simulink model "RM3_Hydraulic_PTO"  (R2019b)
settings: Solver=ode14x  StartTime=0  StopTime=100  FixedStep=0.0025  MaxStep=0.0025  RelTol=1e-3  EnableMultiTasking=on
undefined symbols (not defined in the file or in its folder): body, DiscIntNeverNeededParam, pto
libraries: fl_lib x208, sh_lib x67, nesl_utility x67, WECSim_Lib x5
(part 2 of 5)

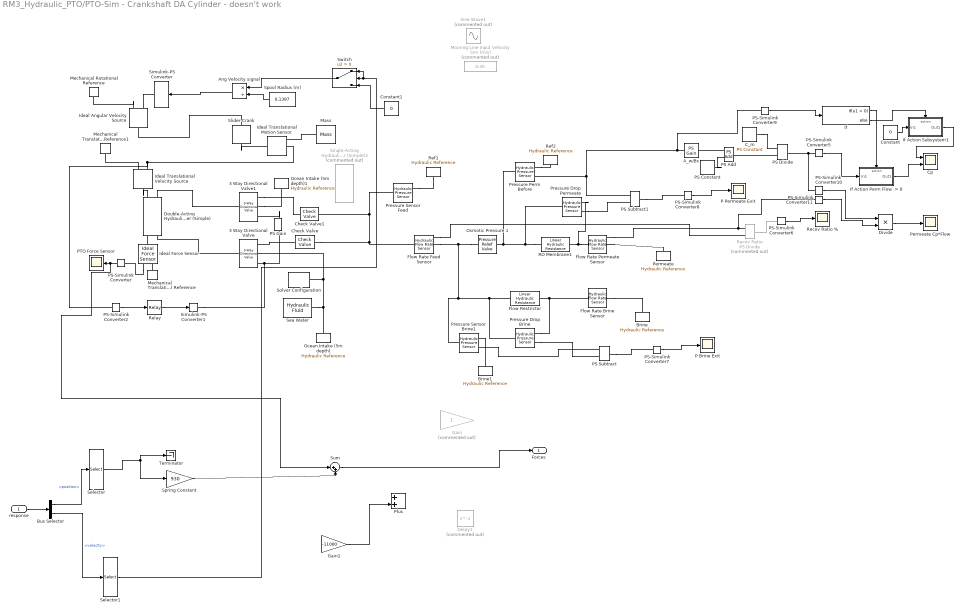
== system RM3_Hydraulic_PTO/PTO-Sim - Crankshaft DA Cylinder - doesn't work ==
  response : Inport
  " Flow Rate Feed Sensor" : fl_lib/Hydraulic/Hydraulic Sensors/Hydraulic Flow Rate Sensor
      settings: SourceProductName=Simscape
  3 Way Directional Valve : sh_lib/Valves/Directional Valves/3-Way Directional Valve  area_spec=sh.valves.directional_valves.enum.area_spec.identical  x_0_P=0 m  x_0_T=0 m  mdl_type_identical=sh.valves.directional_valves.enum.mdl_type.linear  mdl_type_different=sh.valves.directional_valves.enum.mdl_type.linear  opening_max=0.75 in  area_max=pi*(0.75/2)^2 in^2  opening_max_P_A=0.005 m  area_max_P_A=0.5e-4 m^2  opening_max_A_T=0.005 m  area_max_A_T=0.5e-4 m^2  opening_area_tab=[-.002, 0, .002, .005, .015] m  area_tab=[1e-09, 2.0352e-07, 4.0736e-05, .00011438, .00034356] m^2  opening_flow_rate_tab=[-.002, 0, .002, .005, .015] m  pressure_tab=[-10000000, -5000000, -2000000, 2000000, 5000000, 10000000] Pa  flow_rate_tab=[-1e-07, -7.0711e-08, -4.4721e-08, 4.4721e-08, 7.0711e-08, 1e-07; -2.0352e-05, -1.4391e-05, -9.1017e-06, 9.1017e-06, 1.4391e-05, 2.0352e-05; -.0040736, -.0028805, -.0018218, .0018218, .0028805, .0040736; -.011438, -.0080879, -.0051152, .0051152, .0080879, .011438; -.034356, -.024293, -.015364, .015364, .024293, .034356] m^3/s  opening_area_tab_P_A=[-.002, 0, .002, .005, .015] m  area_tab_P_A=[1e-09, 2.0352e-07, 4.0736e-05, .00011438, .00034356] m^2  opening_flow_rate_tab_P_A=[-.002, 0, .002, .005, .015] m  pressure_tab_P_A=[-10000000, -5000000, -2000000, 2000000, 5000000, 10000000] Pa  flow_rate_tab_P_A=[-1e-07, -7.0711e-08, -4.4721e-08, 4.4721e-08, 7.0711e-08, 1e-07; -2.0352e-05, -1.4391e-05, -9.1017e-06, 9.1017e-06, 1.4391e-05, 2.0352e-05; -.0040736, -.0028805, -.0018218, .0018218, .0028805, .0040736; -.011438, -.0080879, -.0051152, .0051152, .0080879, .011438; -.034356, -.024293, -.015364, .015364, .024293, .034356] m^3/s  opening_area_tab_A_T=[-.002, 0, .002, .005, .015] m  area_tab_A_T=[1e-09, 2.0352e-07, 4.0736e-05, .00011438, .00034356] m^2  opening_flow_rate_tab_A_T=[-.002, 0, .002, .005, .015] m  pressure_tab_A_T=[-10000000, -5000000, -2000000, 2000000, 5000000, 10000000] Pa  flow_rate_tab_A_T=[-1e-07, -7.0711e-08, -4.4721e-08, 4.4721e-08, 7.0711e-08, 1e-07; -2.0352e-05, -1.4391e-05, -9.1017e-06, 9.1017e-06, 1.4391e-05, 2.0352e-05; -.0040736, -.0028805, -.0018218, .0018218, .0028805, .0040736; -.011438, -.0080879, -.0051152, .0051152, .0080879, .011438; -.034356, -.024293, -.015364, .015364, .024293, .034356] m^3/s  interp_method_identical=sh.valves.directional_valves.enum.interp_method.linear  interp_method_different=sh.valves.directional_valves.enum.interp_method.linear  extrap_method_identical=sh.valves.directional_valves.enum.extrap_method.linear  extrap_method_different=sh.valves.directional_valves.enum.extrap_method.linear  A_leak=1e-12 m^2  C_d=0.7  lam_spec=sh.valves.directional_valves.enum.lam_spec.pressure_ratio  B_lam=0.999  Re_cr=12
      settings: SourceProductName=Simscape Fluids  SourceProductBaseCode=SH  InternalSimscapePortConfiguration="{\"Bottom\":[],\"Left\":[{\"id\":\"A\",\"label\":\"A\",\"type\":\"foundation.hydraulic.hydraulic\"}],\"Right\":[{\"id\":\"S\",\"label\":\"S\",\"type\":\"input\"},{\"id\":\"P\",\"label\":\"P\",\"type\":\"foundation.hydraulic.hydraulic\"},{\"id\":\"T\",\"label\":\"T\",\"type\":\"foundation.hydraulic.hydraulic\"}],\"Top\":[]}"
  3 Way Directional Valve1 : sh_lib/Valves/Directional Valves/3-Way Directional Valve  area_spec=sh.valves.directional_valves.enum.area_spec.identical  x_0_P=0 m  x_0_T=0 m  mdl_type_identical=sh.valves.directional_valves.enum.mdl_type.linear  mdl_type_different=sh.valves.directional_valves.enum.mdl_type.linear  opening_max=0.75 in  area_max=pi*(0.75/2)^2 in^2  opening_max_P_A=0.005 m  area_max_P_A=0.5e-4 m^2  opening_max_A_T=0.005 m  area_max_A_T=0.5e-4 m^2  opening_area_tab=[-.002, 0, .002, .005, .015] m  area_tab=[1e-09, 2.0352e-07, 4.0736e-05, .00011438, .00034356] m^2  opening_flow_rate_tab=[-.002, 0, .002, .005, .015] m  pressure_tab=[-10000000, -5000000, -2000000, 2000000, 5000000, 10000000] Pa  flow_rate_tab=[-1e-07, -7.0711e-08, -4.4721e-08, 4.4721e-08, 7.0711e-08, 1e-07; -2.0352e-05, -1.4391e-05, -9.1017e-06, 9.1017e-06, 1.4391e-05, 2.0352e-05; -.0040736, -.0028805, -.0018218, .0018218, .0028805, .0040736; -.011438, -.0080879, -.0051152, .0051152, .0080879, .011438; -.034356, -.024293, -.015364, .015364, .024293, .034356] m^3/s  opening_area_tab_P_A=[-.002, 0, .002, .005, .015] m  area_tab_P_A=[1e-09, 2.0352e-07, 4.0736e-05, .00011438, .00034356] m^2  opening_flow_rate_tab_P_A=[-.002, 0, .002, .005, .015] m  pressure_tab_P_A=[-10000000, -5000000, -2000000, 2000000, 5000000, 10000000] Pa  flow_rate_tab_P_A=[-1e-07, -7.0711e-08, -4.4721e-08, 4.4721e-08, 7.0711e-08, 1e-07; -2.0352e-05, -1.4391e-05, -9.1017e-06, 9.1017e-06, 1.4391e-05, 2.0352e-05; -.0040736, -.0028805, -.0018218, .0018218, .0028805, .0040736; -.011438, -.0080879, -.0051152, .0051152, .0080879, .011438; -.034356, -.024293, -.015364, .015364, .024293, .034356] m^3/s  opening_area_tab_A_T=[-.002, 0, .002, .005, .015] m  area_tab_A_T=[1e-09, 2.0352e-07, 4.0736e-05, .00011438, .00034356] m^2  opening_flow_rate_tab_A_T=[-.002, 0, .002, .005, .015] m  pressure_tab_A_T=[-10000000, -5000000, -2000000, 2000000, 5000000, 10000000] Pa  flow_rate_tab_A_T=[-1e-07, -7.0711e-08, -4.4721e-08, 4.4721e-08, 7.0711e-08, 1e-07; -2.0352e-05, -1.4391e-05, -9.1017e-06, 9.1017e-06, 1.4391e-05, 2.0352e-05; -.0040736, -.0028805, -.0018218, .0018218, .0028805, .0040736; -.011438, -.0080879, -.0051152, .0051152, .0080879, .011438; -.034356, -.024293, -.015364, .015364, .024293, .034356] m^3/s  interp_method_identical=sh.valves.directional_valves.enum.interp_method.linear  interp_method_different=sh.valves.directional_valves.enum.interp_method.linear  extrap_method_identical=sh.valves.directional_valves.enum.extrap_method.linear  extrap_method_different=sh.valves.directional_valves.enum.extrap_method.linear  A_leak=1e-12 m^2  C_d=0.7  lam_spec=sh.valves.directional_valves.enum.lam_spec.pressure_ratio  B_lam=0.999  Re_cr=12
      settings: SourceProductName=Simscape Fluids  SourceProductBaseCode=SH  InternalSimscapePortConfiguration="{\"Bottom\":[],\"Left\":[{\"id\":\"A\",\"label\":\"A\",\"type\":\"foundation.hydraulic.hydraulic\"}],\"Right\":[{\"id\":\"S\",\"label\":\"S\",\"type\":\"input\"},{\"id\":\"P\",\"label\":\"P\",\"type\":\"foundation.hydraulic.hydraulic\"},{\"id\":\"T\",\"label\":\"T\",\"type\":\"foundation.hydraulic.hydraulic\"}],\"Top\":[]}"
  A_w/Bs : fl_lib/Physical Signals/Functions/PS Gain  gain=3.812*10^(-12)/(6.986*10^(-8))
  Ang Velocity signal : Product  Inputs=*/
  Brine : fl_lib/Hydraulic/Hydraulic Elements/Hydraulic Reference
      settings: SourceProductName=Simscape
  Brine1 : fl_lib/Hydraulic/Hydraulic Elements/Hydraulic Reference
      settings: SourceProductName=Simscape
  Bus Selector : BusSelector  OutputSignals=position,velocity
  C_m : fl_lib/Physical Signals/Sources/PS Constant  constant=35000
  Check Valve : sh_lib/Valves/Directional Valves/Check Valve  area_max=pi*(0.75/2)^2 in^2  pres_crack=0.3e5 Pa  pres_max=1.2e5 Pa  C_d=0.7  A_leak=1e-12 m^2  lam_spec=1  B_lam=0.999  Re_cr=12  dynamic=0  tau=0.1 s  area_init=1e-12 m^2
      settings: SourceProductName=Simscape Fluids  SourceProductBaseCode=SH  InternalSimscapePortConfiguration="{\"Bottom\":[],\"Left\":[{\"id\":\"A\",\"label\":\"A\",\"type\":\"foundation.hydraulic.hydraulic\"}],\"Right\":[{\"id\":\"B\",\"label\":\"B\",\"type\":\"foundation.hydraulic.hydraulic\"}],\"Top\":[]}"
  Check Valve1 : sh_lib/Valves/Directional Valves/Check Valve  area_max=pi*(0.75/2)^2 in^2  pres_crack=0.3e5 Pa  pres_max=1.2e5 Pa  C_d=0.7  A_leak=1e-12 m^2  lam_spec=1  B_lam=0.999  Re_cr=12  dynamic=0  tau=0.1 s  area_init=1e-12 m^2
      settings: SourceProductName=Simscape Fluids  SourceProductBaseCode=SH  InternalSimscapePortConfiguration="{\"Bottom\":[],\"Left\":[{\"id\":\"A\",\"label\":\"A\",\"type\":\"foundation.hydraulic.hydraulic\"}],\"Right\":[{\"id\":\"B\",\"label\":\"B\",\"type\":\"foundation.hydraulic.hydraulic\"}],\"Top\":[]}"
  Constant : Constant  Value=0
  Constant1 : Constant  Value=0
  Cp : Scope  NumInputPorts=2
  Delay1 : Delay  Commented=on  DelayLength=1
  Divide : Product
  Double-Acting Hydraulic Cylinder (Simple) : sh_lib/Hydraulic Cylinders/Double-Acting Hydraulic Cylinder (Simple)  area_A=0.0025746658 m^2  area_B=0.0025746658 m^2  stroke=12 in  init_pos=5 in  penetr_coeff=1e12 s*N/m^2  or=1
      settings: SourceProductName=Simscape Fluids  SourceProductBaseCode=SH  InternalSimscapePortConfiguration="{\"Bottom\":[],\"Left\":[{\"id\":\"C\",\"label\":\"C\",\"type\":\"foundation.mechanical.translational.translational\"},{\"id\":\"A\",\"label\":\"A\",\"type\":\"foundation.hydraulic.hydraulic\"}],\"Right\":[{\"id\":\"R\",\"label\":\"R\",\"type\":\"foundation.mechanical.translational.translational\"},{\"id\":\"B\",\"label\":\"B\",\"type\":\"foundation.hydraulic.hydraulic\"}],\"Top\":[]}"
  Flow Rate Brine Sensor : fl_lib/Hydraulic/Hydraulic Sensors/Hydraulic Flow Rate Sensor
      settings: SourceProductName=Simscape
  Flow Rate Permeate Sensor : fl_lib/Hydraulic/Hydraulic Sensors/Hydraulic Flow Rate Sensor
      settings: SourceProductName=Simscape
  Flow Restrictor : fl_lib/Hydraulic/Hydraulic Elements/Linear Hydraulic Resistance  resistance=(0.20) * ( 1/((3.812*10^-12)*(7.4 ) ) ) Pa/(m^3/s)  q_specify=off  q_priority=None  q=0.001 m^3/s  q_nominal_specify=off  q_nominal_unit=m^3/s  q_nominal_value=1  p_specify=off  p_priority=None  p=0 Pa  p_nominal_specify=off  p_nominal_unit=Pa  p_nominal_value=1
      settings: SourceProductName=Simscape  SourceProductBaseCode=SS  InternalSimscapePortConfiguration="{\"Bottom\":[],\"Left\":[{\"id\":\"A\",\"label\":\"A\",\"type\":\"foundation.hydraulic.hydraulic\"}],\"Right\":[{\"id\":\"B\",\"label\":\"B\",\"type\":\"foundation.hydraulic.hydraulic\"}],\"Top\":[]}"
  Gain : Gain  Commented=on
  Gain1 : Gain  Gain=-11000
  Ideal Angular Velocity Source : fl_lib/Mechanical/Mechanical Sources/Ideal Angular Velocity Source
  Ideal Force Sensor : fl_lib/Mechanical/Mechanical Sensors/Ideal Force Sensor
  Ideal Translational Motion Sensor : fl_lib/Mechanical/Mechanical Sensors/Ideal Translational Motion Sensor  offset=0 m
  Ideal Translational Velocity Source : fl_lib/Mechanical/Mechanical Sources/Ideal Translational Velocity Source
  If : If
  If Action Perm Flow  > 0 : Subsystem  TreatAsAtomicUnit=on
  If Action Subsystem1 : Subsystem  TreatAsAtomicUnit=on
  Mass : fl_lib/Mechanical/Translational Elements/Mass  mass=1 kg  v_specify=off  v_priority=High  v=0 m/s  v_nominal_specify=off  v_nominal_unit=m/s  v_nominal_value=1  f_specify=off  f_priority=None  f=0 N  f_nominal_specify=off  f_nominal_unit=N  f_nominal_value=1
  Mechanical Rotational Reference : fl_lib/Mechanical/Rotational Elements/Mechanical Rotational Reference
  Mechanical Translational Reference : fl_lib/Mechanical/Translational Elements/Mechanical Translational Reference
  Mechanical Translational Reference1 : fl_lib/Mechanical/Translational Elements/Mechanical Translational Reference
  Mooring Line Input Velocity Sim (m/s) : Constant  Commented=on  Value=0.45
  Ocean Intake (5m depth) : fl_lib/Hydraulic/Hydraulic Elements/Hydraulic Reference
      settings: SourceProductName=Simscape
  Ocean Intake (5m depth)1 : fl_lib/Hydraulic/Hydraulic Elements/Hydraulic Reference
      settings: SourceProductName=Simscape
  Osmotic Pressure 1 : sh_lib/Valves/Pressure Control Valves/Pressure Relief Valve  valve_area_spec=1  p_diff_TLU=[30.15e5 : 15e3 : 31.35e5] Pa  area_TLU=[1 : 1 : 9] .* 1e-5 m^2  area_max=pi*(0.75/2)^2 in^2  pres_set=30 bar  reg_range=2 bar  C_d=0.7  A_leak=1e-12 m^2  lam_spec=1  B_lam=0.999  Re_cr=12  dynamic=0  tau=0.1 s  area_init=1e-12 m^2
      settings: SourceProductName=Simscape Fluids  SourceProductBaseCode=SH  InternalSimscapePortConfiguration="{\"Bottom\":[],\"Left\":[{\"id\":\"A\",\"label\":\"A\",\"type\":\"foundation.hydraulic.hydraulic\"}],\"Right\":[{\"id\":\"B\",\"label\":\"B\",\"type\":\"foundation.hydraulic.hydraulic\"}],\"Top\":[]}"
  P Brine Exit : Scope
  P Permeate Exit : Scope
  PS Add : fl_lib/Physical Signals/Functions/PS Add
  PS Constant : fl_lib/Physical Signals/Sources/PS Constant  constant=1 Pa
  PS Divide : fl_lib/Physical Signals/Functions/PS Divide
      settings: SourceProductName=Simscape  SourceProductBaseCode=SS
  PS Gain : fl_lib/Physical Signals/Functions/PS Gain  gain=-1
  PS Subtract : fl_lib/Physical Signals/Functions/PS Subtract
      settings: SourceProductName=Simscape
  PS Subtract1 : fl_lib/Physical Signals/Functions/PS Subtract
      settings: SourceProductName=Simscape
  PS-Simulink Converter : nesl_utility/PS-Simulink Converter  PhysicalDomain=network_engine_domain  SubClassName=ps_output  LeftPortType=input  RightPortType=output  PseudoPeriodic=off  Frequencies=[]  Unit=N  AffineConversion=off
  PS-Simulink Converter{2,5..11} (8 alike) : nesl_utility/PS-Simulink Converter  PhysicalDomain=network_engine_domain  SubClassName=ps_output  LeftPortType=input  RightPortType=output  PseudoPeriodic=off  Frequencies=[]  Unit=inherit  AffineConversion=off
  PTO Force Sensor : Scope
  Permeate : fl_lib/Hydraulic/Hydraulic Elements/Hydraulic Reference
      settings: SourceProductName=Simscape
  Permeate Cp*Flow : Scope
  Plus : Sum
  Pressure Drop Brine : fl_lib/Hydraulic/Hydraulic Sensors/Hydraulic Pressure Sensor
      settings: SourceProductName=Simscape
  Pressure Drop Permeate : fl_lib/Hydraulic/Hydraulic Sensors/Hydraulic Pressure Sensor
      settings: SourceProductName=Simscape
  Pressure Perm Before : fl_lib/Hydraulic/Hydraulic Sensors/Hydraulic Pressure Sensor
      settings: SourceProductName=Simscape
  Pressure Sensor Brine1 : fl_lib/Hydraulic/Hydraulic Sensors/Hydraulic Pressure Sensor
      settings: SourceProductName=Simscape
  Pressure Sensor Feed : fl_lib/Hydraulic/Hydraulic Sensors/Hydraulic Pressure Sensor
      settings: SourceProductName=Simscape
  RO Membrane1 : fl_lib/Hydraulic/Hydraulic Elements/Linear Hydraulic Resistance  resistance=1/((3.812*10^-12)*(7.4 ) ) Pa/(m^3/s)  q_specify=off  q_priority=None  q=0.001 m^3/s  q_nominal_specify=off  q_nominal_unit=m^3/s  q_nominal_value=1  p_specify=off  p_priority=None  p=0 Pa  p_nominal_specify=off  p_nominal_unit=Pa  p_nominal_value=1
      settings: SourceProductName=Simscape  SourceProductBaseCode=SS  InternalSimscapePortConfiguration="{\"Bottom\":[],\"Left\":[{\"id\":\"A\",\"label\":\"A\",\"type\":\"foundation.hydraulic.hydraulic\"}],\"Right\":[{\"id\":\"B\",\"label\":\"B\",\"type\":\"foundation.hydraulic.hydraulic\"}],\"Top\":[]}"
  Recov Ratio : fl_lib/Physical Signals/Functions/PS Divide  Commented=on
      settings: SourceProductName=Simscape  SourceProductBaseCode=SS
  Recov Ratio % : Scope
  Ref1 : fl_lib/Hydraulic/Hydraulic Elements/Hydraulic Reference
      settings: SourceProductName=Simscape
  Ref2 : fl_lib/Hydraulic/Hydraulic Elements/Hydraulic Reference
      settings: SourceProductName=Simscape
  Relay : Relay  OnSwitchValue=0  OffSwitchValue=0  OffOutputValue=-1
  Sea Water : sh_lib/Hydraulic Utilities/Hydraulic Fluid  DataSource=1  SelFluid=24  SysTemp=30  TrapAir=0.005  ViscDerFactor=1  range_error=2
      settings: SourceProductName=Simscape Fluids
  Selector : Selector  InputPortWidth=6  IndexOptions=Index vector (dialog)  Indices=3  OutputSizes=1
  Selector1 : Selector  InputPortWidth=6  IndexOptions=Index vector (dialog)  Indices=3  OutputSizes=1
  Simulink-PS Converter : nesl_utility/Simulink-PS Converter  PhysicalDomain=network_engine_domain  SubClassName=ps_input  LeftPortType=input  RightPortType=output  PseudoPeriodic=off  Frequencies=[]  NoiseDistribution=none  NoiseParameters=[]  Unit=rad/s  AffineConversion=off  FilteringAndDerivatives=filter  SimscapeFilterOrder=2  InputFilterTimeConstant=0.001  UdotUserProvided=2
  Simulink-PS Converter1 : nesl_utility/Simulink-PS Converter  PhysicalDomain=network_engine_domain  SubClassName=ps_input  LeftPortType=input  RightPortType=output  PseudoPeriodic=off  Frequencies=[]  NoiseDistribution=none  NoiseParameters=[]  Unit=1  AffineConversion=off  FilteringAndDerivatives=zero  SimscapeFilterOrder=1  InputFilterTimeConstant=0.001  UdotUserProvided=0
  Sine Wave1 : Sin  Commented=on  Amplitude=0.45  Frequency=0.9  SampleTime=0.01
  Single-Acting Hydraulic Cylinder (Simple)2 : sh_lib/Hydraulic Cylinders/Single-Acting Hydraulic Cylinder (Simple)  Commented=on  area=0.0025746658 m^2  stroke=12 in  init_pos=0 m  penetr_coeff=1e12 s*N/m^2  or=1
      settings: SourceProductName=Simscape Fluids  SourceProductBaseCode=SH  InternalSimscapePortConfiguration="{\"Bottom\":[],\"Left\":[{\"id\":\"C\",\"label\":\"C\",\"type\":\"foundation.mechanical.translational.translational\"},{\"id\":\"A\",\"label\":\"A\",\"type\":\"foundation.hydraulic.hydraulic\"}],\"Right\":[{\"id\":\"R\",\"label\":\"R\",\"type\":\"foundation.mechanical.translational.translational\"},{\"id\":\"P\",\"label\":\"P\",\"type\":\"output\"}],\"Top\":[]}"
  Slider-Crank : fl_lib/Mechanical/Mechanisms/Slider-Crank  crank=11/2 in  rod=12 in  inertia=0.01 kg*m^2  k=1e6 N/m  b=0.0001 N/(m/s)  theta_specify=off  theta_priority=Low  theta=0 rad  theta_nominal_specify=off  theta_nominal_unit=rad  theta_nominal_value=1  w_specify=off  w_priority=Low  w=0 rad/s  w_nominal_specify=off  w_nominal_unit=rad/s  w_nominal_value=1
      settings: SourceProductName=Simscape  SourceProductBaseCode=SS  InternalSimscapePortConfiguration="{\"Bottom\":[],\"Left\":[{\"id\":\"C\",\"label\":\"C\",\"type\":\"foundation.mechanical.rotational.rotational\"}],\"Right\":[{\"id\":\"S\",\"label\":\"S\",\"type\":\"foundation.mechanical.translational.translational\"}],\"Top\":[]}"
  Solver Configuration : nesl_utility/Solver Configuration  PhysicalDomain=network_engine_domain  SubClassName=solver  LeftPortType=input  RightPortType=generic  Tones=[]  Harmonics=[]  SimulateNoise=off  Profile=off  UseLocalSampling=off  EnableSwitchedLinearOptims=on  FrequencyDomain=off  UseCCode=off  RelTol=0.001  AbsTol=1e-06  MinStep=1e-09  ToWorkspace=off  RevertToSquareIcSolve=off  NumHomotopyIterations=100  PhasorMode=off  PhasorModeNumHarmonics=1  DoDC=off  ResidualTolerance=1e-09  UseLocalSolver=off  LocalSolverChoice=NE_BACKWARD_EULER_ADVANCER  LocalSolverSampleTime=0.001  DoFixedCost=off  MaxNonlinIter=3  MaxModeIter=2  LinearAlgebra=auto  EquationFormulation=NE_TIME_EF  DelaysMemoryBudget=1024  AutomaticFiltering=on  FilteringTimeConstant=0.01  PartitionStorageMethod=AS_NEEDED  PartitionMemoryBudget=1024  PartitionMethod=ROBUST
  Spool Radius (m) : Constant  Value=0.1397
  Spring Constant : Gain  Gain=930
  Sum : Sum  Inputs=|++
  Switch : Switch  Criteria=u2 > Threshold
  Terminator : Terminator
  Forces : Outport  VectorParamsAs1DForOutWhenUnconnected=off
  wires:
  Bus Selector/1 -> Selector/1  "<position>"
  Bus Selector/2 -> Selector1/1  "<velocity>"
  response/1 -> Bus Selector/1
  Selector/1 -> Spring Constant/1, Terminator/1
  Spring Constant/1 -> Sum/2
  Gain1/1 -> Plus/2
  Ang Velocity signal/1 -> Simulink-PS Converter/1
  Constant1/1 -> Switch/3
  If Action Perm Flow  > 0/1(Out1) -> Cp/2
  PS-Simulink Converter2/1 -> Relay/1
  If/1 -> If Action Perm Flow  > 0/Action
  Constant/1 -> If Action Subsystem1/1(In1)
  PS-Simulink Converter/1 -> Sum/1, PTO Force Sensor/1
  Spool Radius (m)/1 -> Ang Velocity signal/2
  If Action Subsystem1/1(Out1) -> Cp/1
  If/2 -> If Action Subsystem1/Action
  PS-Simulink Converter10/1 -> Divide/1
  PS-Simulink Converter5/1 -> If Action Perm Flow  > 0/1(In1)
  PS-Simulink Converter7/1 -> P Brine Exit/1
  Divide/1 -> Permeate Cp*Flow/1
  PS-Simulink Converter8/1 -> P Permeate Exit/1
  Relay/1 -> Simulink-PS Converter1/1
  PS-Simulink Converter11/1 -> Divide/2
  PS-Simulink Converter9/1 -> If/1
  PS-Simulink Converter6/1 -> Recov Ratio %/1
  Sum/1 -> Forces/1
  Selector1/1 -> Switch/1, Switch/2
  Switch/1 -> Ang Velocity signal/1
  connections:
  3 Way Directional Valve/RConn1 -- Simulink-PS Converter1/RConn1 -- PS Gain/LConn1
  Ideal Translational Motion Sensor/RConn2 -- Ideal Translational Velocity Source/RConn1 -- PS-Simulink Converter2/LConn1
  Pressure Perm Before/RConn2 -- A_w/Bs/LConn1 -- PS-Simulink Converter9/LConn1 -- PS Subtract1/LConn1
  Osmotic Pressure 1/LConn1 -- " Flow Rate Feed Sensor"/RConn2 -- Pressure Sensor Brine1/LConn1 -- Pressure Drop Brine/LConn1 -- Flow Restrictor/LConn1
  Flow Restrictor/RConn1 -- Flow Rate Brine Sensor/LConn1 -- Pressure Drop Brine/RConn1
  RO Membrane1/LConn1 -- Pressure Drop Permeate/LConn1 -- Osmotic Pressure 1/RConn1 -- Pressure Perm Before/LConn1
  PS Divide/RConn1 -- PS-Simulink Converter5/LConn1 -- PS-Simulink Converter10/LConn1
  Recov Ratio/LConn1 -- Flow Rate Permeate Sensor/RConn1 -- PS-Simulink Converter11/LConn1
  Flow Rate Permeate Sensor/LConn1 -- RO Membrane1/RConn1 -- Pressure Drop Permeate/RConn1
  Check Valve/RConn1 -- " Flow Rate Feed Sensor"/LConn1 -- Check Valve1/RConn1 -- Pressure Sensor Feed/LConn1
  Solver Configuration/RConn1 -- Sea Water/RConn1 -- Ocean Intake (5m depth)/LConn1 -- 3 Way Directional Valve/RConn2
  Slider-Crank/RConn1 -- Ideal Translational Motion Sensor/LConn1
  Mass/LConn1 -- Ideal Translational Motion Sensor/RConn1
  3 Way Directional Valve1/RConn3 -- Check Valve1/LConn1
  C_m/RConn1 -- PS Divide/LConn1
  PS Add/LConn1 -- A_w/Bs/RConn1
  Pressure Drop Permeate/RConn2 -- PS Subtract1/LConn2
  Slider-Crank/LConn1 -- Ideal Angular Velocity Source/LConn1
  Ideal Angular Velocity Source/RConn1 -- Simulink-PS Converter/RConn1
  PS Subtract/RConn1 -- PS-Simulink Converter7/LConn1
  PS Subtract1/RConn1 -- PS-Simulink Converter8/LConn1
  Ideal Force Sensor/RConn1 -- Mechanical Translational Reference/LConn1
  Recov Ratio/RConn1 -- PS-Simulink Converter6/LConn1
  Pressure Sensor Brine1/RConn1 -- Brine1/LConn1
  " Flow Rate Feed Sensor"/RConn1 -- Recov Ratio/LConn2
  PS Constant/RConn1 -- PS Add/LConn2
  3 Way Directional Valve/LConn1 -- Double-Acting Hydraulic Cylinder (Simple)/LConn2
  Pressure Sensor Feed/RConn1 -- Ref1/LConn1
  Pressure Drop Brine/RConn2 -- PS Subtract/LConn2
  Pressure Perm Before/RConn1 -- Ref2/LConn1
  Ideal Force Sensor/LConn1 -- Double-Acting Hydraulic Cylinder (Simple)/LConn1
  Ideal Force Sensor/RConn2 -- PS-Simulink Converter/LConn1
  PS Gain/RConn1 -- 3 Way Directional Valve1/RConn1
  3 Way Directional Valve1/RConn2 -- Ocean Intake (5m depth)1/LConn1
  PS Divide/LConn2 -- PS Add/RConn1
  Flow Rate Brine Sensor/RConn2 -- Brine/LConn1
  Check Valve/LConn1 -- 3 Way Directional Valve/RConn3
  Ideal Translational Velocity Source/LConn1 -- Double-Acting Hydraulic Cylinder (Simple)/RConn1
  Flow Rate Permeate Sensor/RConn2 -- Permeate/LConn1
  Ideal Angular Velocity Source/RConn2 -- Mechanical Rotational Reference/LConn1
  Ideal Translational Velocity Source/RConn2 -- Mechanical Translational Reference1/LConn1
  Pressure Sensor Brine1/RConn2 -- PS Subtract/LConn1
  Double-Acting Hydraulic Cylinder (Simple)/RConn2 -- 3 Way Directional Valve1/LConn1

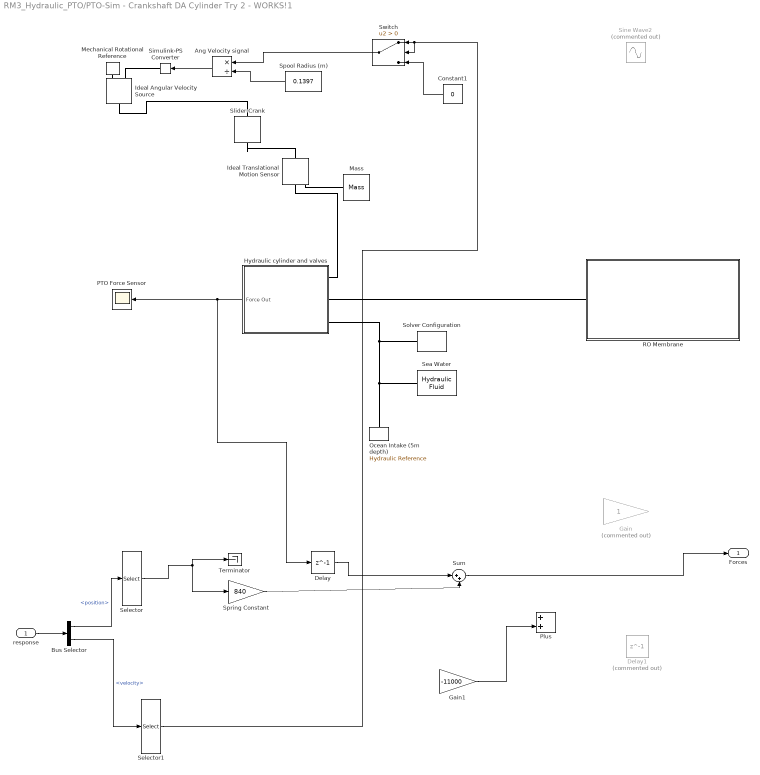
== system RM3_Hydraulic_PTO/PTO-Sim - Crankshaft DA Cylinder Try 2 - WORKS!1 ==
  response : Inport
  Ang Velocity signal : Product  Inputs=*/
  Bus Selector : BusSelector  OutputSignals=position,velocity
  Constant1 : Constant  Value=0
  Delay : Delay  DelayLength=1
  Delay1 : Delay  Commented=on  DelayLength=1
  Gain : Gain  Commented=on
  Gain1 : Gain  Gain=-11000
  Hydraulic cylinder and valves : Subsystem
  Ideal Angular Velocity Source : fl_lib/Mechanical/Mechanical Sources/Ideal Angular Velocity Source
  Ideal Translational Motion Sensor : fl_lib/Mechanical/Mechanical Sensors/Ideal Translational Motion Sensor  offset=0 m
  Mass : fl_lib/Mechanical/Translational Elements/Mass  mass=1 kg  v_specify=off  v_priority=High  v=0 m/s  v_nominal_specify=off  v_nominal_unit=m/s  v_nominal_value=1  f_specify=off  f_priority=None  f=0 N  f_nominal_specify=off  f_nominal_unit=N  f_nominal_value=1
  Mechanical Rotational Reference : fl_lib/Mechanical/Rotational Elements/Mechanical Rotational Reference
  Ocean Intake (5m depth) : fl_lib/Hydraulic/Hydraulic Elements/Hydraulic Reference
      settings: SourceProductName=Simscape
  PTO Force Sensor : Scope
  Plus : Sum
  RO Membrane : Subsystem
  Sea Water : sh_lib/Hydraulic Utilities/Hydraulic Fluid  DataSource=1  SelFluid=24  SysTemp=30  TrapAir=0.005  ViscDerFactor=1  range_error=2
      settings: SourceProductName=Simscape Fluids
  Selector : Selector  InputPortWidth=6  IndexOptions=Index vector (dialog)  Indices=3  OutputSizes=1
  Selector1 : Selector  InputPortWidth=6  IndexOptions=Index vector (dialog)  Indices=3  OutputSizes=1
  Simulink-PS Converter : nesl_utility/Simulink-PS Converter  PhysicalDomain=network_engine_domain  SubClassName=ps_input  LeftPortType=input  RightPortType=output  PseudoPeriodic=off  Frequencies=[]  NoiseDistribution=none  NoiseParameters=[]  Unit=rad/s  AffineConversion=off  FilteringAndDerivatives=filter  SimscapeFilterOrder=2  InputFilterTimeConstant=0.001  UdotUserProvided=0
  Sine Wave2 : Sin  Commented=on  Amplitude=0.45  Frequency=0.9  SampleTime=0.01
  Slider-Crank : fl_lib/Mechanical/Mechanisms/Slider-Crank  crank=11/2 in  rod=12 in  inertia=0.01 kg*m^2  k=1e6 N/m  b=0.0001 N/(m/s)  theta_specify=off  theta_priority=Low  theta=0 rad  theta_nominal_specify=off  theta_nominal_unit=rad  theta_nominal_value=1  w_specify=off  w_priority=Low  w=0 rad/s  w_nominal_specify=off  w_nominal_unit=rad/s  w_nominal_value=1
      settings: SourceProductName=Simscape  SourceProductBaseCode=SS  InternalSimscapePortConfiguration="{\"Bottom\":[],\"Left\":[{\"id\":\"C\",\"label\":\"C\",\"type\":\"foundation.mechanical.rotational.rotational\"}],\"Right\":[{\"id\":\"S\",\"label\":\"S\",\"type\":\"foundation.mechanical.translational.translational\"}],\"Top\":[]}"
  Solver Configuration : nesl_utility/Solver Configuration  PhysicalDomain=network_engine_domain  SubClassName=solver  LeftPortType=input  RightPortType=generic  Tones=[]  Harmonics=[]  SimulateNoise=off  Profile=off  UseLocalSampling=off  EnableSwitchedLinearOptims=on  FrequencyDomain=off  UseCCode=off  RelTol=0.001  AbsTol=1e-06  MinStep=1e-09  ToWorkspace=off  RevertToSquareIcSolve=off  NumHomotopyIterations=100  PhasorMode=off  PhasorModeNumHarmonics=1  DoDC=off  ResidualTolerance=1e-09  UseLocalSolver=off  LocalSolverChoice=NE_BACKWARD_EULER_ADVANCER  LocalSolverSampleTime=0.001  DoFixedCost=off  MaxNonlinIter=3  MaxModeIter=2  LinearAlgebra=auto  EquationFormulation=NE_TIME_EF  DelaysMemoryBudget=1024  AutomaticFiltering=on  FilteringTimeConstant=0.01  PartitionStorageMethod=AS_NEEDED  PartitionMemoryBudget=1024  PartitionMethod=ROBUST
  Spool Radius (m) : Constant  Value=0.1397
  Spring Constant : Gain  Gain=840
  Sum : Sum  Inputs=|++
  Switch : Switch  Criteria=u2 > Threshold
  Terminator : Terminator
  Forces : Outport  VectorParamsAs1DForOutWhenUnconnected=off
  wires:
  Bus Selector/1 -> Selector/1  "<position>"
  Bus Selector/2 -> Selector1/1  "<velocity>"
  response/1 -> Bus Selector/1
  Selector/1 -> Spring Constant/1, Terminator/1
  Spring Constant/1 -> Sum/2
  Gain1/1 -> Plus/2
  Sum/1 -> Forces/1
  Constant1/1 -> Switch/3
  Ang Velocity signal/1 -> Simulink-PS Converter/1
  Switch/1 -> Ang Velocity signal/1
  Hydraulic cylinder and valves/1(Force Out) -> Delay/1, PTO Force Sensor/1
  Spool Radius (m)/1 -> Ang Velocity signal/2
  Selector1/1 -> Switch/2, Switch/1
  Delay/1 -> Sum/1
  connections:
  Solver Configuration/RConn1 -- Hydraulic cylinder and valves/LConn3 -- Ocean Intake (5m depth)/LConn1 -- Sea Water/RConn1
  Hydraulic cylinder and valves/LConn2 -- RO Membrane/LConn1
  Slider-Crank/RConn1 -- Ideal Translational Motion Sensor/LConn1
  Mass/LConn1 -- Ideal Translational Motion Sensor/RConn1
  Ideal Angular Velocity Source/RConn2 -- Mechanical Rotational Reference/LConn1
  Hydraulic cylinder and valves/LConn1 -- Ideal Translational Motion Sensor/RConn2
  Ideal Angular Velocity Source/RConn1 -- Simulink-PS Converter/RConn1
  Slider-Crank/LConn1 -- Ideal Angular Velocity Source/LConn1

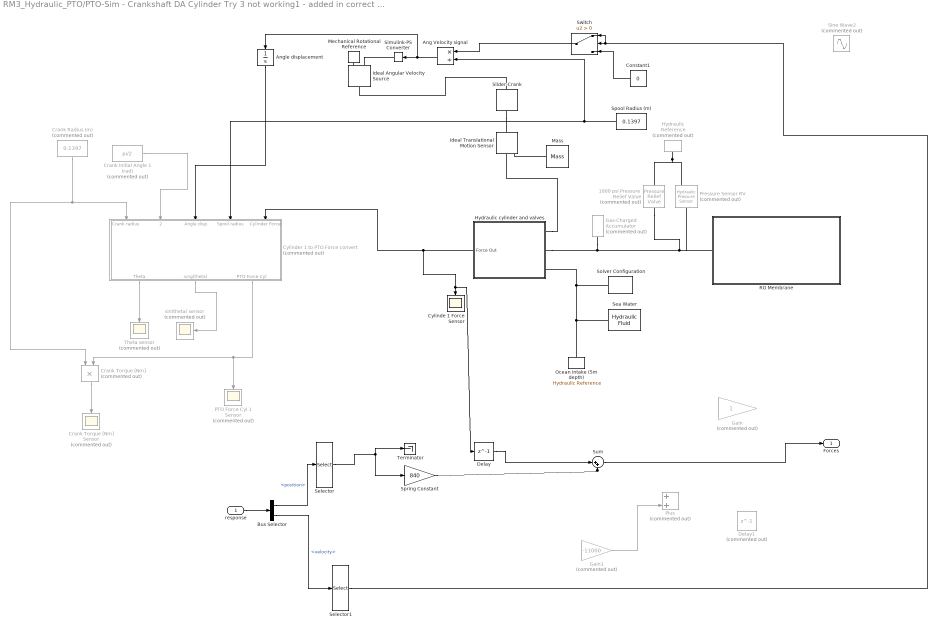
== system RM3_Hydraulic_PTO/PTO-Sim - Crankshaft DA Cylinder Try 3 not working1 - added in correct PTO Force calculation, accumulator, and PR valve ==
  response : Inport
  1000 psi Pressure Relief Valve : sh_lib/Valves/Pressure Control Valves/Pressure Relief Valve  Commented=on  valve_area_spec=1  p_diff_TLU=[30.15e5 : 15e3 : 31.35e5] Pa  area_TLU=[1 : 1 : 9] .* 1e-5 m^2  area_max=pi*(0.75/2)^2 in^2  pres_set=1000 psi  reg_range=50 psi  C_d=0.7  A_leak=1e-12 m^2  lam_spec=1  B_lam=0.999  Re_cr=12  dynamic=0  tau=0.1 s  area_init=1e-12 m^2
      settings: SourceProductName=Simscape Fluids  SourceProductBaseCode=SH  InternalSimscapePortConfiguration="{\"Bottom\":[],\"Left\":[{\"id\":\"A\",\"label\":\"A\",\"type\":\"foundation.hydraulic.hydraulic\"}],\"Right\":[{\"id\":\"B\",\"label\":\"B\",\"type\":\"foundation.hydraulic.hydraulic\"}],\"Top\":[]}"
  Ang Velocity signal : Product  Inputs=*/
  Angle displacement : Integrator
  Bus Selector : BusSelector  OutputSignals=position,velocity
  Constant1 : Constant  Value=0
  Crank Initial Angle 1 (rad) : Constant  Commented=on  Value=pi/2
  Crank Radius (m) : Constant  Commented=on  Value=0.1397
  Crank Torque [Nm] : Product  Commented=on
  Crank Torque [Nm] Sensor : Scope  Commented=on
  Cylinde 1 Force Sensor : Scope
  Cylinder 1 to PTO Force convert : Subsystem  Commented=on
  Delay : Delay  DelayLength=1
  Delay1 : Delay  Commented=on  DelayLength=1
  Gain : Gain  Commented=on
  Gain1 : Gain  Commented=on  Gain=-11000
  Gas-Charged Accumulator : sh_lib/Accumulators/Gas-Charged Accumulator  Commented=on  capacity=2.5 gal  dead_volume=4e-5 m^3  pr_preload=800 psi  k_sh=1.4  stiff_coeff=1e10 Pa/m^3  penetr_coeff=1e10 s*Pa/m^6  flow_rate_specify=off  flow_rate_priority=None  flow_rate=0.005 m^3/s  flow_rate_nominal_specify=off  flow_rate_nominal_unit=m^3/s  flow_rate_nominal_value=1  liquid_volume_specify=on  liquid_volume_priority=High  liquid_volume=0.005 gal  liquid_volume_nominal_specify=off  liquid_volume_nominal_unit=m^3  liquid_volume_nominal_value=1  liquid_pressure_specify=off  liquid_pressure_priority=None  liquid_pressure=1.01325e+5 Pa  liquid_pressure_nominal_specify=off  liquid_pressure_nominal_unit=Pa  liquid_pressure_nominal_value=1
      settings: SourceProductName=Simscape Fluids  SourceProductBaseCode=SH  InternalSimscapePortConfiguration="{\"Bottom\":[],\"Left\":[],\"Right\":[{\"id\":\"A\",\"label\":\"A\",\"type\":\"foundation.hydraulic.hydraulic\"}],\"Top\":[]}"
  Hydraulic Reference : fl_lib/Hydraulic/Hydraulic Elements/Hydraulic Reference  Commented=on
      settings: SourceProductName=Simscape
  Hydraulic cylinder and valves : Subsystem
  Ideal Angular Velocity Source : fl_lib/Mechanical/Mechanical Sources/Ideal Angular Velocity Source
  Ideal Translational Motion Sensor : fl_lib/Mechanical/Mechanical Sensors/Ideal Translational Motion Sensor  offset=0 m
  Mass : fl_lib/Mechanical/Translational Elements/Mass  mass=1 kg  v_specify=off  v_priority=High  v=0 m/s  v_nominal_specify=off  v_nominal_unit=m/s  v_nominal_value=1  f_specify=off  f_priority=None  f=0 N  f_nominal_specify=off  f_nominal_unit=N  f_nominal_value=1
  Mechanical Rotational Reference : fl_lib/Mechanical/Rotational Elements/Mechanical Rotational Reference
  Ocean Intake (5m depth) : fl_lib/Hydraulic/Hydraulic Elements/Hydraulic Reference
      settings: SourceProductName=Simscape
  PTO Force Cyl 1 Sensor : Scope  Commented=on
  Plus : Sum  Commented=on
  Pressure Sensor RV : fl_lib/Hydraulic/Hydraulic Sensors/Hydraulic Pressure Sensor  Commented=on
      settings: SourceProductName=Simscape
  RO Membrane : Subsystem
  Sea Water : sh_lib/Hydraulic Utilities/Hydraulic Fluid  DataSource=1  SelFluid=24  SysTemp=30  TrapAir=0.005  ViscDerFactor=1  range_error=2
      settings: SourceProductName=Simscape Fluids
  Selector : Selector  InputPortWidth=6  IndexOptions=Index vector (dialog)  Indices=3  OutputSizes=1
  Selector1 : Selector  InputPortWidth=6  IndexOptions=Index vector (dialog)  Indices=3  OutputSizes=1
  Simulink-PS Converter : nesl_utility/Simulink-PS Converter  PhysicalDomain=network_engine_domain  SubClassName=ps_input  LeftPortType=input  RightPortType=output  PseudoPeriodic=off  Frequencies=[]  NoiseDistribution=none  NoiseParameters=[]  Unit=rad/s  AffineConversion=off  FilteringAndDerivatives=filter  SimscapeFilterOrder=2  InputFilterTimeConstant=0.001  UdotUserProvided=0
  Sine Wave2 : Sin  Commented=on  Amplitude=0.45  Frequency=0.9  SampleTime=0.01
  Slider-Crank : fl_lib/Mechanical/Mechanisms/Slider-Crank  crank=11/2 in  rod=12 in  inertia=0.01 kg*m^2  k=1e6 N/m  b=0.0001 N/(m/s)  theta_specify=off  theta_priority=Low  theta=0 rad  theta_nominal_specify=off  theta_nominal_unit=rad  theta_nominal_value=1  w_specify=off  w_priority=Low  w=0 rad/s  w_nominal_specify=off  w_nominal_unit=rad/s  w_nominal_value=1
      settings: SourceProductName=Simscape  SourceProductBaseCode=SS  InternalSimscapePortConfiguration="{\"Bottom\":[],\"Left\":[{\"id\":\"C\",\"label\":\"C\",\"type\":\"foundation.mechanical.rotational.rotational\"}],\"Right\":[{\"id\":\"S\",\"label\":\"S\",\"type\":\"foundation.mechanical.translational.translational\"}],\"Top\":[]}"
  Solver Configuration : nesl_utility/Solver Configuration  PhysicalDomain=network_engine_domain  SubClassName=solver  LeftPortType=input  RightPortType=generic  Tones=[]  Harmonics=[]  SimulateNoise=off  Profile=off  UseLocalSampling=off  EnableSwitchedLinearOptims=on  FrequencyDomain=off  UseCCode=off  RelTol=0.001  AbsTol=1e-06  MinStep=1e-09  ToWorkspace=off  RevertToSquareIcSolve=off  NumHomotopyIterations=100  PhasorMode=off  PhasorModeNumHarmonics=1  DoDC=off  ResidualTolerance=1e-09  UseLocalSolver=off  LocalSolverChoice=NE_BACKWARD_EULER_ADVANCER  LocalSolverSampleTime=0.001  DoFixedCost=off  MaxNonlinIter=3  MaxModeIter=2  LinearAlgebra=auto  EquationFormulation=NE_TIME_EF  DelaysMemoryBudget=1024  AutomaticFiltering=on  FilteringTimeConstant=0.01/8  PartitionStorageMethod=AS_NEEDED  PartitionMemoryBudget=1024  PartitionMethod=ROBUST
  Spool Radius (m) : Constant  Value=0.1397
  Spring Constant : Gain  Gain=840
  Sum : Sum  Inputs=|++
  Switch : Switch  Criteria=u2 > Threshold
  Terminator : Terminator
  Theta sensor : Scope  Commented=on
  sin(theta) sensor : Scope  Commented=on
  Forces : Outport  VectorParamsAs1DForOutWhenUnconnected=off
  wires:
  Bus Selector/1 -> Selector/1  "<position>"
  Bus Selector/2 -> Selector1/1  "<velocity>"
  response/1 -> Bus Selector/1
  Selector/1 -> Spring Constant/1, Terminator/1
  Spring Constant/1 -> Sum/2
  Gain1/1 -> Plus/2
  Sum/1 -> Forces/1
  Delay/1 -> Sum/1
  Hydraulic cylinder and valves/1(Force Out) -> Delay/1, Cylinde 1 Force Sensor/1, Cylinder 1 to PTO Force convert/5(Cylinder Force)
  Spool Radius (m)/1 -> Cylinder 1 to PTO Force convert/4(Spool radius), Ang Velocity signal/2
  Ang Velocity signal/1 -> Simulink-PS Converter/1, Angle displacement/1
  Constant1/1 -> Switch/3
  Angle displacement/1 -> Cylinder 1 to PTO Force convert/3(Angle disp)
  Crank Initial Angle 1 (rad)/1 -> Cylinder 1 to PTO Force convert/2(Crank initial angle)
  Crank Torque [Nm]/1 -> Crank Torque [Nm] Sensor/1
  Cylinder 1 to PTO Force convert/1(Theta) -> Theta sensor/1
  Crank Radius (m)/1 -> Crank Torque [Nm]/1, Cylinder 1 to PTO Force convert/1(Crank radius)
  Cylinder 1 to PTO Force convert/2(sing(theta)) -> sin(theta) sensor/1
  Switch/1 -> Ang Velocity signal/1
  Cylinder 1 to PTO Force convert/3(PTO Force Cyl) -> Crank Torque [Nm]/2, PTO Force Cyl 1 Sensor/1
  Selector1/1 -> Switch/1, Switch/2
  connections:
  Sea Water/RConn1 -- Solver Configuration/RConn1 -- Hydraulic cylinder and valves/LConn3 -- Ocean Intake (5m depth)/LConn1
  Hydraulic cylinder and valves/LConn2 -- 1000 psi Pressure Relief Valve/LConn1 -- Pressure Sensor RV/LConn1 -- RO Membrane/LConn1 -- Gas-Charged Accumulator/RConn1
  Hydraulic Reference/LConn1 -- Pressure Sensor RV/RConn1 -- 1000 psi Pressure Relief Valve/RConn1
  Slider-Crank/LConn1 -- Ideal Angular Velocity Source/LConn1
  Mass/LConn1 -- Ideal Translational Motion Sensor/RConn1
  Ideal Angular Velocity Source/RConn1 -- Simulink-PS Converter/RConn1
  Ideal Angular Velocity Source/RConn2 -- Mechanical Rotational Reference/LConn1
  Slider-Crank/RConn1 -- Ideal Translational Motion Sensor/LConn1
  Hydraulic cylinder and valves/LConn1 -- Ideal Translational Motion Sensor/RConn2

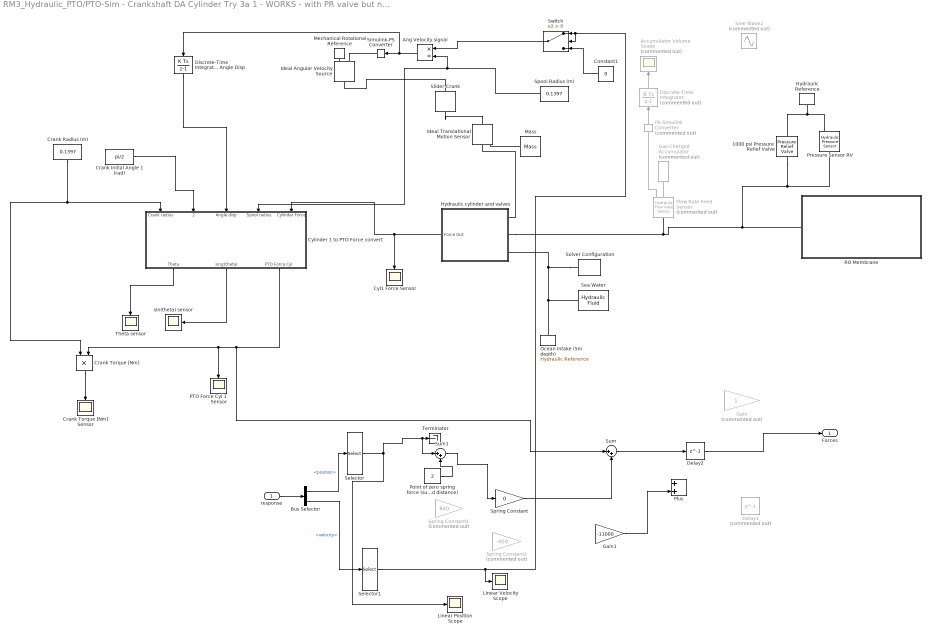
== system RM3_Hydraulic_PTO/PTO-Sim - Crankshaft DA Cylinder Try 3a 1 - WORKS - with PR valve but not ACCUM ==
  response : Inport
  " Flow Rate Feed Sensor" : fl_lib/Hydraulic/Hydraulic Sensors/Hydraulic Flow Rate Sensor  Commented=on
      settings: SourceProductName=Simscape
  1000 psi Pressure Relief Valve : sh_lib/Valves/Pressure Control Valves/Pressure Relief Valve  valve_area_spec=1  p_diff_TLU=[30.15e5 : 15e3 : 31.35e5] Pa  area_TLU=[1 : 1 : 9] .* 1e-5 m^2  area_max=pi*(0.75/2)^2 in^2  pres_set=1000 psi  reg_range=50 psi  C_d=0.7  A_leak=1e-12 m^2  lam_spec=1  B_lam=0.999  Re_cr=12  dynamic=0  tau=0.1 s  area_init=1e-12 m^2
      settings: SourceProductName=Simscape Fluids  SourceProductBaseCode=SH  InternalSimscapePortConfiguration="{\"Bottom\":[],\"Left\":[{\"id\":\"A\",\"label\":\"A\",\"type\":\"foundation.hydraulic.hydraulic\"}],\"Right\":[{\"id\":\"B\",\"label\":\"B\",\"type\":\"foundation.hydraulic.hydraulic\"}],\"Top\":[]}"
  Accumulator Volume Scope : Scope  Commented=on
  Ang Velocity signal : Product  Inputs=*/
  Bus Selector : BusSelector  OutputSignals=position,velocity
  Constant1 : Constant  Value=0
  Crank Initial Angle 1 (rad) : Constant  Value=pi/2
  Crank Radius (m) : Constant  Value=0.1397
  Crank Torque [Nm] : Product
  Crank Torque [Nm] Sensor : Scope
  Cyl1 Force Sensor : Scope
  Cylinder 1 to PTO Force convert : Subsystem
  Delay1 : Delay  Commented=on  DelayLength=1
  Delay2 : Delay  DelayLength=1
  Discrete-Time Integrator : DiscreteIntegrator  Commented=on  SampleTime=-1  ICPrevOutput=DiscIntNeverNeededParam  ICPrevScaledInput=DiscIntNeverNeededParam
  Discrete-Time Integrator - Angle Disp : DiscreteIntegrator  SampleTime=-1  ICPrevOutput=DiscIntNeverNeededParam  ICPrevScaledInput=DiscIntNeverNeededParam
  Gain : Gain  Commented=on
  Gain1 : Gain  Gain=-11000
  Gas-Charged Accumulator : sh_lib/Accumulators/Gas-Charged Accumulator  Commented=on  capacity=2.5 gal  dead_volume=4e-5 m^3  pr_preload=800 psi  k_sh=1.4  stiff_coeff=1e10 Pa/m^3  penetr_coeff=1e10 s*Pa/m^6  flow_rate_specify=on  flow_rate_priority=None  flow_rate=0 m^3/s  flow_rate_nominal_specify=off  flow_rate_nominal_unit=m^3/s  flow_rate_nominal_value=1  liquid_volume_specify=on  liquid_volume_priority=High  liquid_volume=0 gal  liquid_volume_nominal_specify=off  liquid_volume_nominal_unit=m^3  liquid_volume_nominal_value=1  liquid_pressure_specify=off  liquid_pressure_priority=None  liquid_pressure=1.01325e+5 Pa  liquid_pressure_nominal_specify=off  liquid_pressure_nominal_unit=Pa  liquid_pressure_nominal_value=1
      settings: SourceProductName=Simscape Fluids  SourceProductBaseCode=SH  InternalSimscapePortConfiguration="{\"Bottom\":[],\"Left\":[],\"Right\":[{\"id\":\"A\",\"label\":\"A\",\"type\":\"foundation.hydraulic.hydraulic\"}],\"Top\":[]}"
  Hydraulic Reference : fl_lib/Hydraulic/Hydraulic Elements/Hydraulic Reference
      settings: SourceProductName=Simscape
  Hydraulic cylinder and valves : Subsystem
  Ideal Angular Velocity Source : fl_lib/Mechanical/Mechanical Sources/Ideal Angular Velocity Source
  Ideal Translational Motion Sensor : fl_lib/Mechanical/Mechanical Sensors/Ideal Translational Motion Sensor  offset=0 m
  Linear Position Scope : Scope
  Linear Velocity Scope : Scope
  Mass : fl_lib/Mechanical/Translational Elements/Mass  mass=1 kg  v_specify=off  v_priority=High  v=0 m/s  v_nominal_specify=off  v_nominal_unit=m/s  v_nominal_value=1  f_specify=off  f_priority=None  f=0 N  f_nominal_specify=off  f_nominal_unit=N  f_nominal_value=1
  Mechanical Rotational Reference : fl_lib/Mechanical/Rotational Elements/Mechanical Rotational Reference
  Ocean Intake (5m depth) : fl_lib/Hydraulic/Hydraulic Elements/Hydraulic Reference
      settings: SourceProductName=Simscape
  PS-Simulink Converter : nesl_utility/PS-Simulink Converter  Commented=on  PhysicalDomain=network_engine_domain  SubClassName=ps_output  LeftPortType=input  RightPortType=output  PseudoPeriodic=off  Frequencies=[]  Unit=inherit  AffineConversion=off
  PTO Force Cyl 1 Sensor : Scope
  Plus : Sum
  "Point of zero spring force (submerged distance) " : Constant  Value=2
  Pressure Sensor RV : fl_lib/Hydraulic/Hydraulic Sensors/Hydraulic Pressure Sensor
      settings: SourceProductName=Simscape
  RO Membrane : Subsystem
  Sea Water : sh_lib/Hydraulic Utilities/Hydraulic Fluid  DataSource=1  SelFluid=24  SysTemp=30  TrapAir=0.005  ViscDerFactor=1  range_error=2
      settings: SourceProductName=Simscape Fluids
  Selector : Selector  InputPortWidth=6  IndexOptions=Index vector (dialog)  Indices=3  OutputSizes=1
  Selector1 : Selector  InputPortWidth=6  IndexOptions=Index vector (dialog)  Indices=3  OutputSizes=1
  Simulink-PS Converter : nesl_utility/Simulink-PS Converter  PhysicalDomain=network_engine_domain  SubClassName=ps_input  LeftPortType=input  RightPortType=output  PseudoPeriodic=off  Frequencies=[]  NoiseDistribution=none  NoiseParameters=[]  Unit=rad/s  AffineConversion=off  FilteringAndDerivatives=filter  SimscapeFilterOrder=2  InputFilterTimeConstant=0.001  UdotUserProvided=0
  Sine Wave2 : Sin  Commented=on  Amplitude=0.45  Frequency=0.9  SampleTime=0.01
  Slider-Crank : fl_lib/Mechanical/Mechanisms/Slider-Crank  crank=11/2 in  rod=12 in  inertia=0.01 kg*m^2  k=1e6 N/m  b=0.0001 N/(m/s)  theta_specify=off  theta_priority=Low  theta=0 rad  theta_nominal_specify=off  theta_nominal_unit=rad  theta_nominal_value=1  w_specify=off  w_priority=Low  w=0 rad/s  w_nominal_specify=off  w_nominal_unit=rad/s  w_nominal_value=1
      settings: SourceProductName=Simscape  SourceProductBaseCode=SS  InternalSimscapePortConfiguration="{\"Bottom\":[],\"Left\":[{\"id\":\"C\",\"label\":\"C\",\"type\":\"foundation.mechanical.rotational.rotational\"}],\"Right\":[{\"id\":\"S\",\"label\":\"S\",\"type\":\"foundation.mechanical.translational.translational\"}],\"Top\":[]}"
  Solver Configuration : nesl_utility/Solver Configuration  PhysicalDomain=network_engine_domain  SubClassName=solver  LeftPortType=input  RightPortType=generic  Tones=[]  Harmonics=[]  SimulateNoise=off  Profile=off  UseLocalSampling=off  EnableSwitchedLinearOptims=on  FrequencyDomain=off  UseCCode=off  RelTol=0.001  AbsTol=1e-06  MinStep=1e-09  ToWorkspace=off  RevertToSquareIcSolve=off  NumHomotopyIterations=100  PhasorMode=off  PhasorModeNumHarmonics=1  DoDC=off  ResidualTolerance=1e-09  UseLocalSolver=off  LocalSolverChoice=NE_BACKWARD_EULER_ADVANCER  LocalSolverSampleTime=0.001  DoFixedCost=off  MaxNonlinIter=3  MaxModeIter=2  LinearAlgebra=auto  EquationFormulation=NE_TIME_EF  DelaysMemoryBudget=1024  AutomaticFiltering=on  FilteringTimeConstant=0.01  PartitionStorageMethod=AS_NEEDED  PartitionMemoryBudget=1024  PartitionMethod=ROBUST
  Spool Radius (m) : Constant  Value=0.1397
  Spring Constant : Gain  Gain=0
  Spring Constant1 : Gain  Commented=on  Gain=840
  Spring Constant2 : Gain  Commented=on  Gain=-400
  Sum : Sum  Inputs=|++
  Sum1 : Sum  Inputs=|++
  Switch : Switch  Criteria=u2 > Threshold
  Terminator : Terminator
  Theta sensor : Scope
  sin(theta) sensor : Scope
  Forces : Outport  VectorParamsAs1DForOutWhenUnconnected=off
  wires:
  Bus Selector/1 -> Selector/1  "<position>"
  Bus Selector/2 -> Selector1/1  "<velocity>"
  response/1 -> Bus Selector/1
  Selector/1 -> Linear Position Scope/1, Sum1/1, Terminator/1
  Spring Constant/1 -> Sum/2
  Gain1/1 -> Plus/2
  Sum/1 -> Delay2/1
  Constant1/1 -> Switch/3
  Switch/1 -> Ang Velocity signal/1
  Selector1/1 -> Linear Velocity Scope/1, Switch/2, Switch/1
  Cylinder 1 to PTO Force convert/3(PTO Force Cyl) -> Sum/1, Crank Torque [Nm]/2, PTO Force Cyl 1 Sensor/1
  Discrete-Time Integrator - Angle Disp/1 -> Cylinder 1 to PTO Force convert/3(Angle disp)
  Cylinder 1 to PTO Force convert/2(sing(theta)) -> sin(theta) sensor/1
  Cylinder 1 to PTO Force convert/1(Theta) -> Theta sensor/1
  Crank Torque [Nm]/1 -> Crank Torque [Nm] Sensor/1
  Crank Initial Angle 1 (rad)/1 -> Cylinder 1 to PTO Force convert/2(Crank initial angle)
  Crank Radius (m)/1 -> Crank Torque [Nm]/1, Cylinder 1 to PTO Force convert/1(Crank radius)
  Spool Radius (m)/1 -> Cylinder 1 to PTO Force convert/4(Spool radius), Ang Velocity signal/2
  Hydraulic cylinder and valves/1(Force Out) -> Cylinder 1 to PTO Force convert/5(Cylinder Force), Cyl1 Force Sensor/1
  Ang Velocity signal/1 -> Discrete-Time Integrator - Angle Disp/1, Simulink-PS Converter/1
  "Point of zero spring force (submerged distance) "/1 -> Sum1/2
  Sum1/1 -> Spring Constant/1
  Delay2/1 -> Forces/1
  PS-Simulink Converter/1 -> Discrete-Time Integrator/1
  Discrete-Time Integrator/1 -> Accumulator Volume Scope/1
  connections:
  Solver Configuration/RConn1 -- Hydraulic cylinder and valves/LConn3 -- Ocean Intake (5m depth)/LConn1 -- Sea Water/RConn1
  Slider-Crank/RConn1 -- Ideal Translational Motion Sensor/LConn1
  Mass/LConn1 -- Ideal Translational Motion Sensor/RConn1
  Ideal Angular Velocity Source/RConn2 -- Mechanical Rotational Reference/LConn1
  Hydraulic cylinder and valves/LConn1 -- Ideal Translational Motion Sensor/RConn2
  Ideal Angular Velocity Source/RConn1 -- Simulink-PS Converter/RConn1
  Slider-Crank/LConn1 -- Ideal Angular Velocity Source/LConn1
  1000 psi Pressure Relief Valve/RConn1 -- Pressure Sensor RV/RConn1 -- Hydraulic Reference/LConn1
  Hydraulic cylinder and valves/LConn2 -- 1000 psi Pressure Relief Valve/LConn1 -- Pressure Sensor RV/LConn1 -- RO Membrane/LConn1 -- " Flow Rate Feed Sensor"/LConn1
  " Flow Rate Feed Sensor"/RConn2 -- Gas-Charged Accumulator/RConn1
  " Flow Rate Feed Sensor"/RConn1 -- PS-Simulink Converter/LConn1

== system RM3_Hydraulic_PTO/PTO-Sim - Crankshaft DA 4 Cylinders Try 4 WORKS /Cylinder 1 ==
  Crank Radius : Inport
  Spool Radius : Inport  Port=2
  Angle Displacement : Inport  Port=3
  Crank Init Angle : Inport  Port=4
  Crank Torque [Nm] : Product
  Crank Torque [Nm] Sensor : Scope
  Cyl1 Force Sensor : Scope
  Cylinder 1 to PTO Force convert : Subsystem
  Hydraulic cylinder and valves : Subsystem
  Ideal Translational Motion Sensor : fl_lib/Mechanical/Mechanical Sensors/Ideal Translational Motion Sensor  offset=0 m
  Mass : fl_lib/Mechanical/Translational Elements/Mass  mass=1 kg  v_specify=off  v_priority=High  v=0 m/s  v_nominal_specify=off  v_nominal_unit=m/s  v_nominal_value=1  f_specify=off  f_priority=None  f=0 N  f_nominal_specify=off  f_nominal_unit=N  f_nominal_value=1
  PTO Force Cyl 1 Sensor : Scope
  Slider-Crank : fl_lib/Mechanical/Mechanisms/Slider-Crank  crank=11/2 in  rod=12 in  inertia=0.01 kg*m^2  k=1e6 N/m  b=0.0001 N/(m/s)  theta_specify=on  theta_priority=High  theta=pi / 2 rad  theta_nominal_specify=off  theta_nominal_unit=rad  theta_nominal_value=1  w_specify=off  w_priority=Low  w=0 rad/s  w_nominal_specify=off  w_nominal_unit=rad/s  w_nominal_value=1
      settings: SourceProductName=Simscape  SourceProductBaseCode=SS  InternalSimscapePortConfiguration="{\"Bottom\":[],\"Left\":[{\"id\":\"C\",\"label\":\"C\",\"type\":\"foundation.mechanical.rotational.rotational\"}],\"Right\":[{\"id\":\"S\",\"label\":\"S\",\"type\":\"foundation.mechanical.translational.translational\"}],\"Top\":[]}"
  Theta sensor : Scope
  sin(theta) sensor : Scope
  Angular Vel Source : PMIOPort  Side=Left
  Flow Out : PMIOPort  Port=2  Side=Left
  Flow In : PMIOPort  Port=3  Side=Left
  PTO Force : Outport
  wires:
  Crank Torque [Nm]/1 -> Crank Torque [Nm] Sensor/1
  Hydraulic cylinder and valves/1(Force Out) -> Cylinder 1 to PTO Force convert/5(Cylinder Force), Cyl1 Force Sensor/1
  Crank Radius/1 -> Cylinder 1 to PTO Force convert/1(Crank radius), Crank Torque [Nm]/1
  Cylinder 1 to PTO Force convert/3(PTO Force Cyl) -> PTO Force/1, Crank Torque [Nm]/2, PTO Force Cyl 1 Sensor/1
  Cylinder 1 to PTO Force convert/2(sing(theta)) -> sin(theta) sensor/1
  Spool Radius/1 -> Cylinder 1 to PTO Force convert/4(Spool radius)
  Cylinder 1 to PTO Force convert/1(Theta) -> Theta sensor/1
  Crank Init Angle/1 -> Cylinder 1 to PTO Force convert/2(Crank initial angle)
  Angle Displacement/1 -> Cylinder 1 to PTO Force convert/3(Angle disp)
  connections:
  Hydraulic cylinder and valves/LConn1 -- Ideal Translational Motion Sensor/RConn2
  Mass/LConn1 -- Ideal Translational Motion Sensor/RConn1
  Slider-Crank/RConn1 -- Ideal Translational Motion Sensor/LConn1
  Slider-Crank/LConn1 -- Angular Vel Source/RConn1
  Flow In/RConn1 -- Hydraulic cylinder and valves/LConn3
  Hydraulic cylinder and valves/LConn2 -- Flow Out/RConn1
